simulink library "minionLogic"  (R2014b)
settings: Solver=ode45  StartTime=0.0  StopTime=10.0  RelTol=1e-3
settings Model: Creator=scastro  LastModifiedBy=scastro

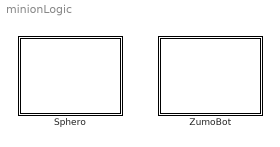
== system minionLogic ==
  Sphero : Stateflow chart  TreatAsAtomicUnit=on
  ZumoBot : Stateflow chart  TreatAsAtomicUnit=on

== stateflow chart minionLogic/ZumoBot ==
  note: ZumoBot related logic
  state Standby
  (default) -> Standby

== stateflow chart minionLogic/Sphero ==
  note: Sphero related logic
  state Standby
  (default) -> Standby
